simulink model "start"  (R2017b)
settings: Solver=VariableStepAuto  StartTime=0.0  StopTime=20  RelTol=1e-3
undefined symbols (not defined in the file or in its folder): m, r
libraries: simulink x1
settings Model: Creator=Administrator  LastModifiedBy=Administrator
settings DataIOCC: Refine=5

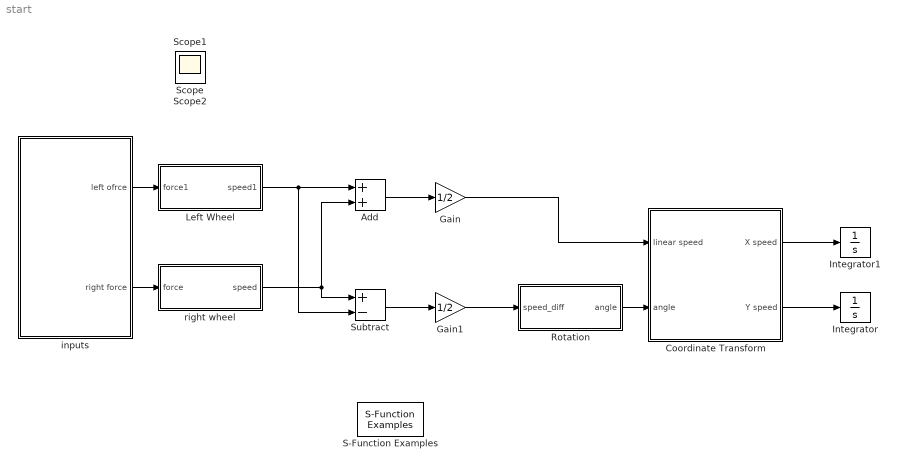
== system start ==
  Add : Sum
  Coordinate Transform : Subsystem
  Gain : Gain  Gain=1/2
  Gain1 : Gain  Gain=1/2
  Integrator : Integrator
  Integrator1 : Integrator
  Left Wheel : Subsystem
  Rotation : Subsystem
  S-Function Examples : simulink/User-Defined Functions/S-Function Examples
      settings: SourceProductName=Simulink  SourceProductBaseCode=SL
  Subtract : Sum  Inputs=+-
  inputs : Subsystem
  right wheel : Subsystem
  Scope : Scope
  Scope1 : Scope
  Scope2 : Scope
  wires:
  right wheel/1(speed) -> Subtract/1, Add/2
  Add/1 -> Gain/1
  Subtract/1 -> Gain1/1
  inputs/2(right force) -> right wheel/1(force)
  Gain1/1 -> Rotation/1(speed_diff)
  Rotation/1(angle) -> Coordinate Transform/2(angle)
  Coordinate Transform/1(X speed) -> Integrator1/1
  Coordinate Transform/2(Y speed) -> Integrator/1
  Gain/1 -> Coordinate Transform/1(linear speed)
  inputs/1(left ofrce) -> Left Wheel/1(force1)
  Left Wheel/1(speed1) -> Subtract/2, Add/1

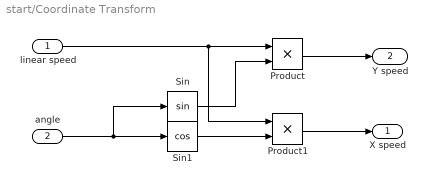
== system start/Coordinate Transform ==
  linear speed : Inport
  angle : Inport  Port=2
  Product : Product
  Product1 : Product
  Sin : Trigonometry
  Sin1 : Trigonometry  Operator=cos
  X speed : Outport
  Y speed : Outport  Port=2
  wires:
  angle/1 -> Sin/1, Sin1/1
  linear speed/1 -> Product1/1, Product/1
  Sin/1 -> Product/2
  Sin1/1 -> Product1/2
  Product1/1 -> X speed/1
  Product/1 -> Y speed/1

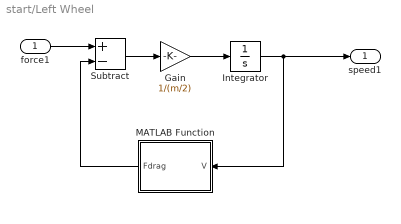
== system start/Left Wheel ==
  force1 : Inport
  Gain : Gain  Gain=1/(m/2)
  Integrator : Integrator
  MATLAB Function : MATLAB Function  TreatAsAtomicUnit=on
  Subtract : Sum  Inputs=+-
  speed1 : Outport
  wires:
  force1/1 -> Subtract/1
  MATLAB Function/1(Fdrag) -> Subtract/2
  Gain/1 -> Integrator/1
  Subtract/1 -> Gain/1
  Integrator/1 -> MATLAB Function/1(V), speed1/1

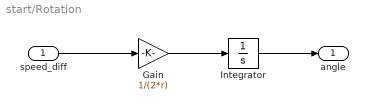
== system start/Rotation ==
  speed_diff : Inport
  Gain : Gain  Gain=1/(2*r)
  Integrator : Integrator  InitialCondition=pi/4
  angle : Outport
  wires:
  speed_diff/1 -> Gain/1
  Gain/1 -> Integrator/1
  Integrator/1 -> angle/1

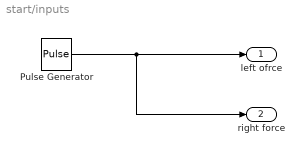
== system start/inputs ==
  Pulse Generator : DiscretePulseGenerator  PulseType=Time based  Period=20  PulseWidth=15
  left ofrce : Outport
  right force : Outport  Port=2
  wires:
  Pulse Generator/1 -> right force/1, left ofrce/1

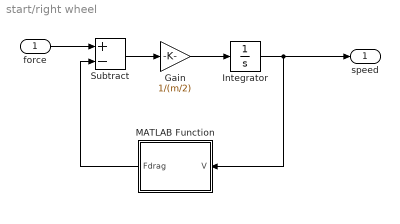
== system start/right wheel ==
  force : Inport
  Gain : Gain  Gain=1/(m/2)
  Integrator : Integrator
  MATLAB Function : MATLAB Function  TreatAsAtomicUnit=on
  Subtract : Sum  Inputs=+-
  speed : Outport
  wires:
  Integrator/1 -> MATLAB Function/1(V), speed/1
  force/1 -> Subtract/1
  MATLAB Function/1(Fdrag) -> Subtract/2
  Subtract/1 -> Gain/1
  Gain/1 -> Integrator/1

== matlab function start/Left Wheel/MATLAB Function ==
  data: V input; Fdrag output; K_drag parameter
function Fdrag = get_fdrag(V,K_drag)    

Fdrag = K_drag*V*abs(V);

== matlab function start/right wheel/MATLAB Function ==
  data: V input; Fdrag output; K_drag parameter
function Fdrag = get_fdrag(V,K_drag)    

Fdrag = K_drag*V*abs(V);
